simulink model "Demo_veDYNA_cs"  (Simulink 7.6)
settings: Solver=ode1  StartTime=0  StopTime=15  FixedStep=1/500  RelTol=1e-3
PreLoadFcn:
  | PreScanveDYNAPreLoadFcn(bdroot);
  | check_NUTS_defined;
  | 
  | assignin('base',['model_closed_' bdroot],false);
PostLoadFcn:
  | PreScanveDYNAPostLoadFcn(bdroot);
  | 
InitFcn:
  | vdy_SetExternalInputSource('ManLongCtrl',1,'Brake','other');
  | vdy_SetExternalInputSource('ManLongCtrl',1,'EngineTorque','other');
  | vdy_SetExternalInputSource('ManLatCtrl',1,'Steering','other');
  | 
  | PreScanveDYNAInitFcn(bdroot);
  | PreScanExperimentInitFcn(bdroot)
StopFcn:
  | PreScanExperimentStopFcn(bdroot)
undefined symbols (not defined in the file): at_period, CPT, vm_at_pulsewidth, vm_driver_dflt_gain, x_ini_VRML, y_ini_VRML, z_ini_VRML
libraries: dyna_cpt_lib x93, simulink x16, simulink_extras x14, PreScanSimulinkLibrary x6, anilib x3, dyna_lib x3, dyna_manctrl_lib x2, dyna_road_lib x2, PreScanUsefulBlocks x1, dyna_io_lib x1, dyna_demo_lib x1, dyna_usr_maneuver_states_lib x1
(part 6 of 8)

== system Demo_veDYNA_cs/Vedyna_Vehicle/CPT_MDL/MDL_SW/GearCtrl/System Instance 1 ==
  Gear [1,..,4] : Subsystem
      mask Display: disp('Input switch: value(1), table(2), io(3), other(4) [1,..,4]')
  GearMode [0,1] : Subsystem
      mask Display: disp('Input switch: internal(0), external(1) [0,1]')
  HCI [1,..,n] : Subsystem
      mask Display: disp('HCI switch [1,..,n]')
  UpShiftRequest [1,..,4] : Subsystem
      mask Display: disp('Input switch: value(1), table(2), io(3), other(4) [1,..,4]')

== system Demo_veDYNA_cs/Vedyna_Vehicle/CPT_MDL/MDL_SW/ManLatCtrl/System Instance 1 ==
  Curvature [1,..,4] : Subsystem
      mask Display: disp('Input switch: value(1), table(2), io(3), other(4) [1,..,4]')
  LatManMode [0,1,2] : Subsystem
      mask Display: disp('Input switch: internal(0), ext. steering(1), ext. curvature(2) [0,1,2]')
  Steering [1,..,4] : Subsystem
      mask Display: disp('Input switch: value(1), table(2), io(3), other(4) [1,..,4]')

== system Demo_veDYNA_cs/Vedyna_Vehicle/CPT_MDL/MDL_SW/ManLongCtrl/System Instance 1 ==
  AccelerationY [1,..,4] : Subsystem
      mask Display: disp('Input switch: value(1), table(2), io(3), other(4) [1,..,4]')
  Brake [1,..,4] : Subsystem
      mask Display: disp('Input switch: value(1), table(2), io(3), other(4) [1,..,4]')
  EngineTorque [1,..,4] : Subsystem
      mask Display: disp('Input switch: value(1), table(2), io(3), other(4) [1,..,4]')
  LongManMode [0,1,2] : Subsystem
      mask Display: disp('Input switch: internal(0), ext. throttle/brake(1), ext. speed(2) [0,1,2]')
  Speed [1,..,4] : Subsystem
      mask Display: disp('Input switch: value(1), table(2), io(3), other(4) [1,..,4]')
  Throttle [1,..,4] : Subsystem
      mask Display: disp('Input switch: value(1), table(2), io(3), other(4) [1,..,4]')

== system Demo_veDYNA_cs/Vedyna_Vehicle/CPT_MDL/MDL_SW/ManSchedule/System Instance 1 ==
  HCI [1,..,n] : Subsystem
      mask Display: disp('HCI switch [1,..,n]')

== system Demo_veDYNA_cs/Vedyna_Vehicle/CPT_MDL/MDL_SW/ManSchedule/System Instance 2 ==
  HCI [1,..,n] : Subsystem
      mask Display: disp('HCI switch [1,..,n]')

== system Demo_veDYNA_cs/Vedyna_Vehicle/CPT_MDL/MDL_SW/ManSchedule/System Instance 3 ==
  HCI [1,..,n] : Subsystem
      mask Display: disp('HCI switch [1,..,n]')

== system Demo_veDYNA_cs/Vedyna_Vehicle/CPT_MDL/MDL_SW/Road/System Instance 1 ==
  HCI [1,..,n] : Subsystem
      mask Display: disp('HCI switch [1,..,n]')

== system Demo_veDYNA_cs/Vedyna_Vehicle/CPT_MDL/MDL_SW/Simctrl/System Instance 1 ==
  Reset [0,1] : Subsystem
      mask Display: disp('Reset switch: 0/1 [0,1]')
  Suspend [0,1] : Subsystem
      mask Display: disp('Suspend switch: 0/1 [0,1]')

== system Demo_veDYNA_cs/Vedyna_Vehicle/CPT_MDL/MDL_SW/Tmeasy/System Instance 1 ==
  HCI [1,..,n] : Subsystem
      mask Display: disp('HCI switch [1,..,n]')
  RoadMueScale [1,..,4] : Subsystem
      mask Display: disp('Input switch: value(1), table(2), io(3), other(4) [1,..,4]')

== system Demo_veDYNA_cs/Vedyna_Vehicle/CPT_MDL/MDL_SW/Tmeasy/System Instance 2 ==
  HCI [1,..,n] : Subsystem
      mask Display: disp('HCI switch [1,..,n]')
  RoadMueScale [1,..,4] : Subsystem
      mask Display: disp('Input switch: value(1), table(2), io(3), other(4) [1,..,4]')

== system Demo_veDYNA_cs/Vedyna_Vehicle/CPT_MDL/MDL_SW/Tmeasy/System Instance 3 ==
  HCI [1,..,n] : Subsystem
      mask Display: disp('HCI switch [1,..,n]')
  RoadMueScale [1,..,4] : Subsystem
      mask Display: disp('Input switch: value(1), table(2), io(3), other(4) [1,..,4]')

== system Demo_veDYNA_cs/Vedyna_Vehicle/CPT_MDL/MDL_SW/Tmeasy/System Instance 4 ==
  HCI [1,..,n] : Subsystem
      mask Display: disp('HCI switch [1,..,n]')
  RoadMueScale [1,..,4] : Subsystem
      mask Display: disp('Input switch: value(1), table(2), io(3), other(4) [1,..,4]')

== system Demo_veDYNA_cs/Vedyna_Vehicle/CPT_MDL/MDL_SW/Tmeasy/System Instance 5 ==
  HCI [1,..,n] : Subsystem
      mask Display: disp('HCI switch [1,..,n]')
  RoadMueScale [1,..,4] : Subsystem
      mask Display: disp('Input switch: value(1), table(2), io(3), other(4) [1,..,4]')

== system Demo_veDYNA_cs/Vedyna_Vehicle/CPT_MDL/MDL_SW/Tmeasy/System Instance 6 ==
  HCI [1,..,n] : Subsystem
      mask Display: disp('HCI switch [1,..,n]')
  RoadMueScale [1,..,4] : Subsystem
      mask Display: disp('Input switch: value(1), table(2), io(3), other(4) [1,..,4]')

== system Demo_veDYNA_cs/Vedyna_Vehicle/CPT_MDL/MDL_SW/Tmeasy/System Instance 7 ==
  HCI [1,..,n] : Subsystem
      mask Display: disp('HCI switch [1,..,n]')
  RoadMueScale [1,..,4] : Subsystem
      mask Display: disp('Input switch: value(1), table(2), io(3), other(4) [1,..,4]')

== system Demo_veDYNA_cs/Vedyna_Vehicle/CPT_MDL/MDL_SW/Tmeasy/System Instance 8 ==
  HCI [1,..,n] : Subsystem
      mask Display: disp('HCI switch [1,..,n]')
  RoadMueScale [1,..,4] : Subsystem
      mask Display: disp('Input switch: value(1), table(2), io(3), other(4) [1,..,4]')

== system Demo_veDYNA_cs/Vedyna_Vehicle/CPT_MDL/MDL_SW/Vehicle/System Instance 1 ==
  HCI [1,..,n] : Subsystem
      mask Display: disp('HCI switch [1,..,n]')

== system Demo_veDYNA_cs/Vedyna_Vehicle/CPT_MDL/MDL_SW/Wheel/System Instance 1 ==
  HCI [1,..,n] : Subsystem
      mask Display: disp('HCI switch [1,..,n]')
  pbrm [1,..,4] : Subsystem
      mask Display: disp('Input switch: value(1), table(2), io(3), other(4) [1,..,4]')

== system Demo_veDYNA_cs/Vedyna_Vehicle/CPT_MDL/MDL_SW/Wheel/System Instance 2 ==
  HCI [1,..,n] : Subsystem
      mask Display: disp('HCI switch [1,..,n]')
  pbrm [1,..,4] : Subsystem
      mask Display: disp('Input switch: value(1), table(2), io(3), other(4) [1,..,4]')

== system Demo_veDYNA_cs/Vedyna_Vehicle/CPT_MDL/MDL_SW/Wheel/System Instance 3 ==
  HCI [1,..,n] : Subsystem
      mask Display: disp('HCI switch [1,..,n]')
  pbrm [1,..,4] : Subsystem
      mask Display: disp('Input switch: value(1), table(2), io(3), other(4) [1,..,4]')

== system Demo_veDYNA_cs/Vedyna_Vehicle/CPT_MDL/MDL_SW/Wheel/System Instance 4 ==
  HCI [1,..,n] : Subsystem
      mask Display: disp('HCI switch [1,..,n]')
  pbrm [1,..,4] : Subsystem
      mask Display: disp('Input switch: value(1), table(2), io(3), other(4) [1,..,4]')

== system Demo_veDYNA_cs/Vedyna_Vehicle/CPT_MDL/MDL_SW/Wheel/System Instance 5 ==
  HCI [1,..,n] : Subsystem
      mask Display: disp('HCI switch [1,..,n]')
  pbrm [1,..,4] : Subsystem
      mask Display: disp('Input switch: value(1), table(2), io(3), other(4) [1,..,4]')

== system Demo_veDYNA_cs/Vedyna_Vehicle/CPT_MDL/MDL_SW/Wheel/System Instance 6 ==
  HCI [1,..,n] : Subsystem
      mask Display: disp('HCI switch [1,..,n]')
  pbrm [1,..,4] : Subsystem
      mask Display: disp('Input switch: value(1), table(2), io(3), other(4) [1,..,4]')

== system Demo_veDYNA_cs/Vedyna_Vehicle/CPT_MDL/MDL_SW/Wheel/System Instance 7 ==
  HCI [1,..,n] : Subsystem
      mask Display: disp('HCI switch [1,..,n]')
  pbrm [1,..,4] : Subsystem
      mask Display: disp('Input switch: value(1), table(2), io(3), other(4) [1,..,4]')

== system Demo_veDYNA_cs/Vedyna_Vehicle/CPT_MDL/MDL_SW/Wheel/System Instance 8 ==
  HCI [1,..,n] : Subsystem
      mask Display: disp('HCI switch [1,..,n]')
  pbrm [1,..,4] : Subsystem
      mask Display: disp('Input switch: value(1), table(2), io(3), other(4) [1,..,4]')

== system Demo_veDYNA_cs/Vedyna_Vehicle/vdy_mdl/Maneuver Control/Maneuver Controller Inputs/Clutch Control Inputs ==
  Ground : Ground
  Ground1 : Ground
  Mux : Mux  Inputs=2
  PAR_ClutchCtrl_1_Clutch : dyna_cpt_lib/CPT_MDL_PAR_ACCESS  Tag=vedynaCPT_MDL_PAR_ACCESS  component=ClutchCtrl  system_inst=1  parameter=Clutch
  SW_ClutchCtrl_1_ClutchMode : dyna_cpt_lib/CPT_MDL_SW_ACCESS  Tag=vedynaCPT_MDL_HCI_ACCESS  component=ClutchCtrl  system_inst=1  parameter=ClutchMode
  Scale to [0..1] : Gain  Gain=0.01  SaturateOnIntegerOverflow=on  OutDataTypeStr=Inherit: Same as input  ParamDataTypeStr=Inherit: Same as input
  Clutch Control Inputs : Outport
  wires:
  Scale to [0..1]/1 -> Mux/2
  PAR_ClutchCtrl_1_Clutch/1 -> Scale to [0..1]/1
  Ground1/1 -> PAR_ClutchCtrl_1_Clutch/1
  Ground/1 -> PAR_ClutchCtrl_1_Clutch/2
  SW_ClutchCtrl_1_ClutchMode/1 -> Mux/1
  Mux/1 -> Clutch Control Inputs/1

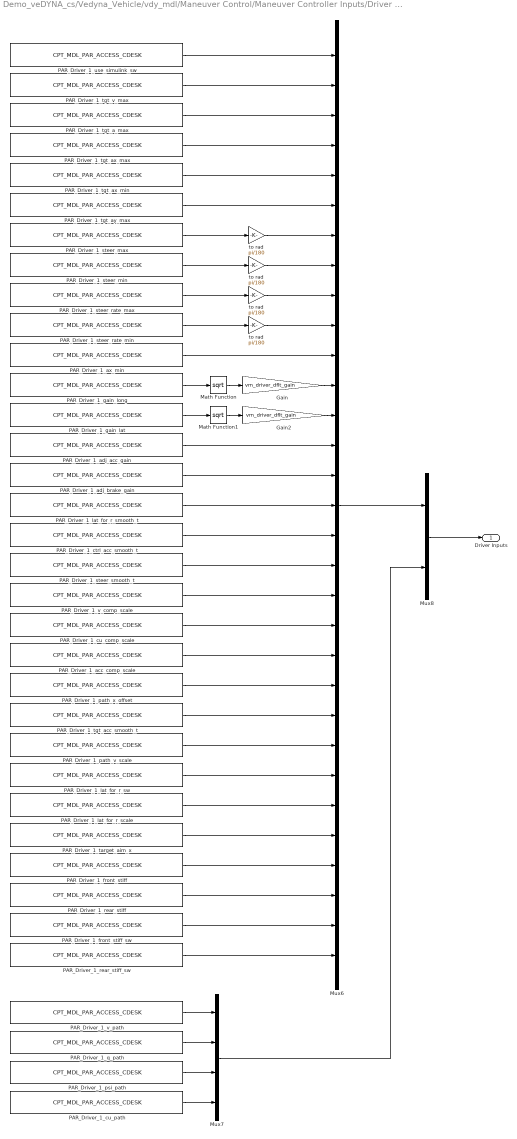
== system Demo_veDYNA_cs/Vedyna_Vehicle/vdy_mdl/Maneuver Control/Maneuver Controller Inputs/Driver Inputs ==
  Gain : Gain  Gain=vm_driver_dflt_gain  SaturateOnIntegerOverflow=on  OutDataTypeStr=Inherit: Same as input  ParamDataTypeStr=Inherit: Same as input
  Gain2 : Gain  Gain=vm_driver_dflt_gain  SaturateOnIntegerOverflow=on  OutDataTypeStr=Inherit: Same as input  ParamDataTypeStr=Inherit: Same as input
  Math Function : Math  Operator=sqrt  SaturateOnIntegerOverflow=on
  Math Function1 : Math  Operator=sqrt  SaturateOnIntegerOverflow=on
  Mux6 : Mux  Inputs=31
  Mux7 : Mux
  Mux8 : Mux  Inputs=2
  PAR_Driver_1_acc_comp_scale : dyna_cpt_lib/CPT_MDL_PAR_ACCESS_CDESK  Tag=vedynaCPT_MDL_PAR_ACCESS  component=Driver  system_inst=1  parameter=acc_comp_scale
  PAR_Driver_1_adj_acc_gain : dyna_cpt_lib/CPT_MDL_PAR_ACCESS_CDESK  Tag=vedynaCPT_MDL_PAR_ACCESS  component=Driver  system_inst=1  parameter=adj_acc_gain
  PAR_Driver_1_adj_brake_gain : dyna_cpt_lib/CPT_MDL_PAR_ACCESS_CDESK  Tag=vedynaCPT_MDL_PAR_ACCESS  component=Driver  system_inst=1  parameter=adj_brake_gain
  PAR_Driver_1_ax_min : dyna_cpt_lib/CPT_MDL_PAR_ACCESS_CDESK  Tag=vedynaCPT_MDL_PAR_ACCESS  component=Driver  system_inst=1  parameter=ax_min
  PAR_Driver_1_ctrl_acc_smooth_t : dyna_cpt_lib/CPT_MDL_PAR_ACCESS_CDESK  Tag=vedynaCPT_MDL_PAR_ACCESS  component=Driver  system_inst=1  parameter=ctrl_acc_smooth_t
  PAR_Driver_1_cu_comp_scale : dyna_cpt_lib/CPT_MDL_PAR_ACCESS_CDESK  Tag=vedynaCPT_MDL_PAR_ACCESS  component=Driver  system_inst=1  parameter=cu_comp_scale
  PAR_Driver_1_cu_path : dyna_cpt_lib/CPT_MDL_PAR_ACCESS_CDESK  Tag=vedynaCPT_MDL_PAR_ACCESS  component=Driver  system_inst=1  parameter=cu_path
  PAR_Driver_1_front_stiff : dyna_cpt_lib/CPT_MDL_PAR_ACCESS_CDESK  Tag=vedynaCPT_MDL_PAR_ACCESS  component=Driver  system_inst=1  parameter=front_stiff
  PAR_Driver_1_front_stiff_sw : dyna_cpt_lib/CPT_MDL_PAR_ACCESS_CDESK  Tag=vedynaCPT_MDL_PAR_ACCESS  component=Driver  system_inst=1  parameter=front_stiff_sw
  PAR_Driver_1_gain_lat : dyna_cpt_lib/CPT_MDL_PAR_ACCESS_CDESK  Tag=vedynaCPT_MDL_PAR_ACCESS  component=Driver  system_inst=1  parameter=gain_lat
  PAR_Driver_1_gain_long : dyna_cpt_lib/CPT_MDL_PAR_ACCESS_CDESK  Tag=vedynaCPT_MDL_PAR_ACCESS  component=Driver  system_inst=1  parameter=gain_long
  PAR_Driver_1_lat_for_r_scale : dyna_cpt_lib/CPT_MDL_PAR_ACCESS_CDESK  Tag=vedynaCPT_MDL_PAR_ACCESS  component=Driver  system_inst=1  parameter=lat_for_r_scale
  PAR_Driver_1_lat_for_r_smooth_t : dyna_cpt_lib/CPT_MDL_PAR_ACCESS_CDESK  Tag=vedynaCPT_MDL_PAR_ACCESS  component=Driver  system_inst=1  parameter=lat_for_r_smooth_t
  PAR_Driver_1_lat_for_r_sw : dyna_cpt_lib/CPT_MDL_PAR_ACCESS_CDESK  Tag=vedynaCPT_MDL_PAR_ACCESS  component=Driver  system_inst=1  parameter=lat_for_r_sw
  PAR_Driver_1_path_v_scale : dyna_cpt_lib/CPT_MDL_PAR_ACCESS_CDESK  Tag=vedynaCPT_MDL_PAR_ACCESS  component=Driver  system_inst=1  parameter=path_v_scale
  PAR_Driver_1_path_x_offset : dyna_cpt_lib/CPT_MDL_PAR_ACCESS_CDESK  Tag=vedynaCPT_MDL_PAR_ACCESS  component=Driver  system_inst=1  parameter=path_x_offset
  PAR_Driver_1_psi_path : dyna_cpt_lib/CPT_MDL_PAR_ACCESS_CDESK  Tag=vedynaCPT_MDL_PAR_ACCESS  component=Driver  system_inst=1  parameter=psi_path
  PAR_Driver_1_q_path : dyna_cpt_lib/CPT_MDL_PAR_ACCESS_CDESK  Tag=vedynaCPT_MDL_PAR_ACCESS  component=Driver  system_inst=1  parameter=q_path
  PAR_Driver_1_rear_stiff : dyna_cpt_lib/CPT_MDL_PAR_ACCESS_CDESK  Tag=vedynaCPT_MDL_PAR_ACCESS  component=Driver  system_inst=1  parameter=rear_stiff
  PAR_Driver_1_rear_stiff_sw : dyna_cpt_lib/CPT_MDL_PAR_ACCESS_CDESK  Tag=vedynaCPT_MDL_PAR_ACCESS  component=Driver  system_inst=1  parameter=rear_stiff_sw
  PAR_Driver_1_steer_max : dyna_cpt_lib/CPT_MDL_PAR_ACCESS_CDESK  Tag=vedynaCPT_MDL_PAR_ACCESS  component=Driver  system_inst=1  parameter=steer_max
  PAR_Driver_1_steer_min : dyna_cpt_lib/CPT_MDL_PAR_ACCESS_CDESK  Tag=vedynaCPT_MDL_PAR_ACCESS  component=Driver  system_inst=1  parameter=steer_min
  PAR_Driver_1_steer_rate_max : dyna_cpt_lib/CPT_MDL_PAR_ACCESS_CDESK  Tag=vedynaCPT_MDL_PAR_ACCESS  component=Driver  system_inst=1  parameter=steer_rate_max
  PAR_Driver_1_steer_rate_min : dyna_cpt_lib/CPT_MDL_PAR_ACCESS_CDESK  Tag=vedynaCPT_MDL_PAR_ACCESS  component=Driver  system_inst=1  parameter=steer_rate_min
  PAR_Driver_1_steer_smooth_t : dyna_cpt_lib/CPT_MDL_PAR_ACCESS_CDESK  Tag=vedynaCPT_MDL_PAR_ACCESS  component=Driver  system_inst=1  parameter=steer_smooth_t
  PAR_Driver_1_target_aim_x : dyna_cpt_lib/CPT_MDL_PAR_ACCESS_CDESK  Tag=vedynaCPT_MDL_PAR_ACCESS  component=Driver  system_inst=1  parameter=target_aim_x
  PAR_Driver_1_tgt_a_max : dyna_cpt_lib/CPT_MDL_PAR_ACCESS_CDESK  Tag=vedynaCPT_MDL_PAR_ACCESS  component=Driver  system_inst=1  parameter=tgt_a_max
  PAR_Driver_1_tgt_acc_smooth_t : dyna_cpt_lib/CPT_MDL_PAR_ACCESS_CDESK  Tag=vedynaCPT_MDL_PAR_ACCESS  component=Driver  system_inst=1  parameter=tgt_acc_smooth_t
  PAR_Driver_1_tgt_ax_max : dyna_cpt_lib/CPT_MDL_PAR_ACCESS_CDESK  Tag=vedynaCPT_MDL_PAR_ACCESS  component=Driver  system_inst=1  parameter=tgt_ax_max
  PAR_Driver_1_tgt_ax_min : dyna_cpt_lib/CPT_MDL_PAR_ACCESS_CDESK  Tag=vedynaCPT_MDL_PAR_ACCESS  component=Driver  system_inst=1  parameter=tgt_ax_min
  PAR_Driver_1_tgt_ay_max : dyna_cpt_lib/CPT_MDL_PAR_ACCESS_CDESK  Tag=vedynaCPT_MDL_PAR_ACCESS  component=Driver  system_inst=1  parameter=tgt_ay_max
  PAR_Driver_1_tgt_v_max : dyna_cpt_lib/CPT_MDL_PAR_ACCESS_CDESK  Tag=vedynaCPT_MDL_PAR_ACCESS  component=Driver  system_inst=1  parameter=tgt_v_max
  PAR_Driver_1_use_simulink_sw : dyna_cpt_lib/CPT_MDL_PAR_ACCESS_CDESK  Tag=vedynaCPT_MDL_PAR_ACCESS  component=Driver  system_inst=1  parameter=use_simulink_sw
  PAR_Driver_1_v_comp_scale : dyna_cpt_lib/CPT_MDL_PAR_ACCESS_CDESK  Tag=vedynaCPT_MDL_PAR_ACCESS  component=Driver  system_inst=1  parameter=v_comp_scale
  PAR_Driver_1_v_path : dyna_cpt_lib/CPT_MDL_PAR_ACCESS_CDESK  Tag=vedynaCPT_MDL_PAR_ACCESS  component=Driver  system_inst=1  parameter=v_path
  to rad : Gain  Gain=pi/180  SaturateOnIntegerOverflow=on  OutDataTypeStr=Inherit: Same as input  ParamDataTypeStr=Inherit: Same as input
  "to rad " : Gain  Gain=pi/180  SaturateOnIntegerOverflow=on  OutDataTypeStr=Inherit: Same as input  ParamDataTypeStr=Inherit: Same as input
  "to rad  " : Gain  Gain=pi/180  SaturateOnIntegerOverflow=on  OutDataTypeStr=Inherit: Same as input  ParamDataTypeStr=Inherit: Same as input
  "to rad   " : Gain  Gain=pi/180  SaturateOnIntegerOverflow=on  OutDataTypeStr=Inherit: Same as input  ParamDataTypeStr=Inherit: Same as input
  Driver Inputs : Outport
  wires:
  to rad/1 -> Mux6/7
  PAR_Driver_1_steer_max/1 -> to rad/1
  "to rad "/1 -> Mux6/8
  PAR_Driver_1_steer_min/1 -> "to rad "/1
  "to rad  "/1 -> Mux6/9
  PAR_Driver_1_steer_rate_max/1 -> "to rad  "/1
  "to rad   "/1 -> Mux6/10
  PAR_Driver_1_steer_rate_min/1 -> "to rad   "/1
  Math Function1/1 -> Gain2/1
  PAR_Driver_1_gain_lat/1 -> Math Function1/1
  Math Function/1 -> Gain/1
  PAR_Driver_1_gain_long/1 -> Math Function/1
  Gain2/1 -> Mux6/13
  Gain/1 -> Mux6/12
  Mux7/1 -> Mux8/2
  Mux8/1 -> Driver Inputs/1
  Mux6/1 -> Mux8/1
  PAR_Driver_1_cu_path/1 -> Mux7/4
  PAR_Driver_1_psi_path/1 -> Mux7/3
  PAR_Driver_1_q_path/1 -> Mux7/2
  PAR_Driver_1_v_path/1 -> Mux7/1
  PAR_Driver_1_rear_stiff_sw/1 -> Mux6/31
  PAR_Driver_1_front_stiff_sw/1 -> Mux6/30
  PAR_Driver_1_rear_stiff/1 -> Mux6/29
  PAR_Driver_1_front_stiff/1 -> Mux6/28
  PAR_Driver_1_target_aim_x/1 -> Mux6/27
  PAR_Driver_1_lat_for_r_scale/1 -> Mux6/26
  PAR_Driver_1_lat_for_r_sw/1 -> Mux6/25
  PAR_Driver_1_path_v_scale/1 -> Mux6/24
  PAR_Driver_1_tgt_acc_smooth_t/1 -> Mux6/23
  PAR_Driver_1_path_x_offset/1 -> Mux6/22
  PAR_Driver_1_acc_comp_scale/1 -> Mux6/21
  PAR_Driver_1_cu_comp_scale/1 -> Mux6/20
  PAR_Driver_1_v_comp_scale/1 -> Mux6/19
  PAR_Driver_1_steer_smooth_t/1 -> Mux6/18
  PAR_Driver_1_ctrl_acc_smooth_t/1 -> Mux6/17
  PAR_Driver_1_lat_for_r_smooth_t/1 -> Mux6/16
  PAR_Driver_1_adj_brake_gain/1 -> Mux6/15
  PAR_Driver_1_adj_acc_gain/1 -> Mux6/14
  PAR_Driver_1_ax_min/1 -> Mux6/11
  PAR_Driver_1_tgt_ay_max/1 -> Mux6/6
  PAR_Driver_1_tgt_ax_min/1 -> Mux6/5
  PAR_Driver_1_tgt_ax_max/1 -> Mux6/4
  PAR_Driver_1_tgt_a_max/1 -> Mux6/3
  PAR_Driver_1_tgt_v_max/1 -> Mux6/2
  PAR_Driver_1_use_simulink_sw/1 -> Mux6/1

== system Demo_veDYNA_cs/Vedyna_Vehicle/vdy_mdl/Maneuver Control/Maneuver Controller Inputs/Gear Control Inputs ==
  Ground{,1..3} (4 alike) : Ground
  Mux : Mux  Inputs=3
  PAR_GearCtrl_1_Gear : dyna_cpt_lib/CPT_MDL_PAR_ACCESS  Tag=vedynaCPT_MDL_PAR_ACCESS  component=GearCtrl  system_inst=1  parameter=Gear
  PAR_GearCtrl_1_UpShiftRequest : dyna_cpt_lib/CPT_MDL_PAR_ACCESS  Tag=vedynaCPT_MDL_PAR_ACCESS  component=GearCtrl  system_inst=1  parameter=UpShiftRequest
  SW_GearCtrl_1_GearMode : dyna_cpt_lib/CPT_MDL_SW_ACCESS  Tag=vedynaCPT_MDL_HCI_ACCESS  component=GearCtrl  system_inst=1  parameter=GearMode
  Gear Control Inputs : Outport
  wires:
  Ground1/1 -> PAR_GearCtrl_1_Gear/1
  Ground/1 -> PAR_GearCtrl_1_Gear/2
  SW_GearCtrl_1_GearMode/1 -> Mux/1
  PAR_GearCtrl_1_Gear/1 -> Mux/2
  PAR_GearCtrl_1_UpShiftRequest/1 -> Mux/3
  Ground3/1 -> PAR_GearCtrl_1_UpShiftRequest/1
  Ground2/1 -> PAR_GearCtrl_1_UpShiftRequest/2
  Mux/1 -> Gear Control Inputs/1

== system Demo_veDYNA_cs/Vedyna_Vehicle/vdy_mdl/Maneuver Control/Maneuver Controller Inputs/Lateral Control Inputs ==
  Ground{,1..3} (4 alike) : Ground
  Mux : Mux  Inputs=3
  PAR_ManLatCtrl_1_Curvature : dyna_cpt_lib/CPT_MDL_PAR_ACCESS  Tag=vedynaCPT_MDL_PAR_ACCESS  component=ManLatCtrl  system_inst=1  parameter=Curvature
  PAR_ManLatCtrl_1_Steering : dyna_cpt_lib/CPT_MDL_PAR_ACCESS  Tag=vedynaCPT_MDL_PAR_ACCESS  component=ManLatCtrl  system_inst=1  parameter=Steering
  SW_ManLatCtrl_1_LatManMode : dyna_cpt_lib/CPT_MDL_SW_ACCESS  Tag=vedynaCPT_MDL_HCI_ACCESS  component=ManLatCtrl  system_inst=1  parameter=LatManMode
  Scale to [rad] : Gain  Gain=pi/180  SaturateOnIntegerOverflow=on  OutDataTypeStr=Inherit: Same as input  ParamDataTypeStr=Inherit: Same as input
  Lateral Control Inputs : Outport
  wires:
  Scale to [rad]/1 -> Mux/2
  PAR_ManLatCtrl_1_Steering/1 -> Scale to [rad]/1
  SW_ManLatCtrl_1_LatManMode/1 -> Mux/1
  PAR_ManLatCtrl_1_Curvature/1 -> Mux/3
  Ground1/1 -> PAR_ManLatCtrl_1_Steering/1
  Ground/1 -> PAR_ManLatCtrl_1_Steering/2
  Ground3/1 -> PAR_ManLatCtrl_1_Curvature/1
  Ground2/1 -> PAR_ManLatCtrl_1_Curvature/2
  Mux/1 -> Lateral Control Inputs/1

== system Demo_veDYNA_cs/Vedyna_Vehicle/vdy_mdl/Maneuver Control/Maneuver Controller Inputs/Longitudinal Control Inputs ==
  Ground{,1..9} (10 alike) : Ground
  Mux : Mux  Inputs=6
  PAR_ManLongCtrl_1_AccelerationY : dyna_cpt_lib/CPT_MDL_PAR_ACCESS  Tag=vedynaCPT_MDL_PAR_ACCESS  component=ManLongCtrl  system_inst=1  parameter=AccelerationY
  PAR_ManLongCtrl_1_Brake : dyna_cpt_lib/CPT_MDL_PAR_ACCESS  Tag=vedynaCPT_MDL_PAR_ACCESS  component=ManLongCtrl  system_inst=1  parameter=Brake
  PAR_ManLongCtrl_1_EngineTorque : dyna_cpt_lib/CPT_MDL_PAR_ACCESS  Tag=vedynaCPT_MDL_PAR_ACCESS  component=ManLongCtrl  system_inst=1  parameter=EngineTorque
  PAR_ManLongCtrl_1_Speed : dyna_cpt_lib/CPT_MDL_PAR_ACCESS  Tag=vedynaCPT_MDL_PAR_ACCESS  component=ManLongCtrl  system_inst=1  parameter=Speed
  PAR_ManLongCtrl_1_Throttle : dyna_cpt_lib/CPT_MDL_PAR_ACCESS  Tag=vedynaCPT_MDL_PAR_ACCESS  component=ManLongCtrl  system_inst=1  parameter=Throttle
  SW_ManLongCtrl_1_LongManMode : dyna_cpt_lib/CPT_MDL_SW_ACCESS  Tag=vedynaCPT_MDL_HCI_ACCESS  component=ManLongCtrl  system_inst=1  parameter=LongManMode
  Scale to [0..1] : Gain  Gain=0.01  SaturateOnIntegerOverflow=on  OutDataTypeStr=Inherit: Same as input  ParamDataTypeStr=Inherit: Same as input
  Scale to [0..1]1 : Gain  Gain=0.01  SaturateOnIntegerOverflow=on  OutDataTypeStr=Inherit: Same as input  ParamDataTypeStr=Inherit: Same as input
  Scale to [m/s] : Gain  Gain=1/3.6  SaturateOnIntegerOverflow=on  OutDataTypeStr=Inherit: Same as input  ParamDataTypeStr=Inherit: Same as input
  Longitudinal Control Inputs : Outport
  wires:
  Scale to [m/s]/1 -> Mux/5
  PAR_ManLongCtrl_1_Speed/1 -> Scale to [m/s]/1
  Scale to [0..1]1/1 -> Mux/3
  PAR_ManLongCtrl_1_Brake/1 -> Scale to [0..1]1/1
  Scale to [0..1]/1 -> Mux/2
  PAR_ManLongCtrl_1_Throttle/1 -> Scale to [0..1]/1
  Ground1/1 -> PAR_ManLongCtrl_1_Throttle/1
  Ground/1 -> PAR_ManLongCtrl_1_Throttle/2
  SW_ManLongCtrl_1_LongManMode/1 -> Mux/1
  PAR_ManLongCtrl_1_AccelerationY/1 -> Mux/4
  PAR_ManLongCtrl_1_EngineTorque/1 -> Mux/6
  Ground9/1 -> PAR_ManLongCtrl_1_EngineTorque/1
  Ground8/1 -> PAR_ManLongCtrl_1_EngineTorque/2
  Ground7/1 -> PAR_ManLongCtrl_1_Speed/1
  Ground6/1 -> PAR_ManLongCtrl_1_Speed/2
  Ground5/1 -> PAR_ManLongCtrl_1_AccelerationY/1
  Ground4/1 -> PAR_ManLongCtrl_1_AccelerationY/2
  Ground3/1 -> PAR_ManLongCtrl_1_Brake/1
  Ground2/1 -> PAR_ManLongCtrl_1_Brake/2
  Mux/1 -> Longitudinal Control Inputs/1

== system Demo_veDYNA_cs/Vedyna_Vehicle/vdy_mdl/Road/veDYNA Road Subsystem/HCI Switch ==
  SW_Road_1_HCI : dyna_cpt_lib/CPT_MDL_HCI_SW_ACCESS  Tag=vedynaCPT_MDL_HCI_SW_ACCESS  component=Road  system_inst=1  parameter=HCI
  HCI Switch : Outport
  wires:
  SW_Road_1_HCI/1 -> HCI Switch/1

== system Demo_veDYNA_cs/Vedyna_Vehicle/vdy_mdl/Vehicle System/veDYNA Vehicle Subsystem/Brake System ==
  note: COPYRIGHT 2004 by TESIS DYNAware GmbH
  note: veDYNA Vehicle Brake System
  SyncIn : Inport
  I/O Vector : Inport  Port=2
  Brake Pedal Position : Inport  Port=3
  Configurable Subsystem : Subsystem  BlockChoice=veDYNA Brake Hydraulics
      settings: AttributesFormatString=%<BlockChoice>  MemberBlocks=User Defined Brake Hydraulics,veDYNA Brake Hydraulics,veDYNA Brake Hydraulics Trailer
      settings: TemplateBlock=|
      | dyna_brakehydraulics_lib/Configurable
      | Subsystem
  Constant{,1..5} (6 alike) : Constant  Value=0
  HCI Switch : Subsystem
  Mux1 : Mux  Inputs=6
  PAR_Wheel_1_pbrm : dyna_cpt_lib/CPT_MDL_PAR_ACCESS  Tag=vedynaCPT_MDL_PAR_ACCESS  component=Wheel  system_inst=1  parameter=pbrm
  PAR_Wheel_2_pbrm : dyna_cpt_lib/CPT_MDL_PAR_ACCESS  Tag=vedynaCPT_MDL_PAR_ACCESS  component=Wheel  system_inst=2  parameter=pbrm
  PAR_Wheel_3_pbrm : dyna_cpt_lib/CPT_MDL_PAR_ACCESS  Tag=vedynaCPT_MDL_PAR_ACCESS  component=Wheel  system_inst=3  parameter=pbrm
  PAR_Wheel_4_pbrm : dyna_cpt_lib/CPT_MDL_PAR_ACCESS  Tag=vedynaCPT_MDL_PAR_ACCESS  component=Wheel  system_inst=4  parameter=pbrm
  PAR_Wheel_5_pbrm : dyna_cpt_lib/CPT_MDL_PAR_ACCESS  Tag=vedynaCPT_MDL_PAR_ACCESS  component=Wheel  system_inst=5  parameter=pbrm
  PAR_Wheel_6_pbrm : dyna_cpt_lib/CPT_MDL_PAR_ACCESS  Tag=vedynaCPT_MDL_PAR_ACCESS  component=Wheel  system_inst=6  parameter=pbrm
  Terminator10 : Terminator
  Terminator4 : Terminator
  Brake Hydraulics Info : Outport
  SyncOut : Outport  Port=2
  Master Cylinder Pressure : Outport  Port=3
  Wheel Cylinder Pressures : Outport  Port=4
  tag scope: pb=global, pbmax=global
  wires:
  Configurable Subsystem/11(Wheel 8 Cylinder Pressure) -> Terminator10/1
  Configurable Subsystem/10(Wheel 7 Cylinder Pressure) -> Terminator4/1
  I/O Vector/1 -> Configurable Subsystem/2(I/O Vector)
  PAR_Wheel_2_pbrm/1 -> Mux1/2
  PAR_Wheel_3_pbrm/1 -> Mux1/3
  PAR_Wheel_4_pbrm/1 -> Mux1/4
  Mux1/1 -> Wheel Cylinder Pressures/1
  SyncIn/1 -> Configurable Subsystem/3(SyncIn)
  Brake Pedal Position/1 -> Configurable Subsystem/1(Brake Pedal Position)
  PAR_Wheel_1_pbrm/1 -> Mux1/1
  Configurable Subsystem/1(SyncOut) -> SyncOut/1
  Configurable Subsystem/2(BrkHyd Info) -> Brake Hydraulics Info/1, [pbmax]
  Configurable Subsystem/3(Master Cylinder Pressure) -> Master Cylinder Pressure/1, [pb]
  PAR_Wheel_5_pbrm/1 -> Mux1/5
  PAR_Wheel_6_pbrm/1 -> Mux1/6
  HCI Switch/1(HCI Switch) -> Configurable Subsystem/4(HCI Switch)
  Constant/1 -> PAR_Wheel_1_pbrm/1
  Configurable Subsystem/4(Wheel 1 Cylinder Pressure) -> PAR_Wheel_1_pbrm/2
  Configurable Subsystem/5(Wheel 2 Cylinder Pressure) -> PAR_Wheel_2_pbrm/2
  Configurable Subsystem/6(Wheel 3 Cylinder Pressure) -> PAR_Wheel_3_pbrm/2
  Configurable Subsystem/7(Wheel 4 Cylinder Pressure) -> PAR_Wheel_4_pbrm/2
  Configurable Subsystem/8(Wheel 5 Cylinder Pressure) -> PAR_Wheel_5_pbrm/2
  Configurable Subsystem/9(Wheel 6 Cylinder Pressure) -> PAR_Wheel_6_pbrm/2
  Constant1/1 -> PAR_Wheel_2_pbrm/1
  Constant2/1 -> PAR_Wheel_3_pbrm/1
  Constant3/1 -> PAR_Wheel_4_pbrm/1
  Constant4/1 -> PAR_Wheel_5_pbrm/1
  Constant5/1 -> PAR_Wheel_6_pbrm/1

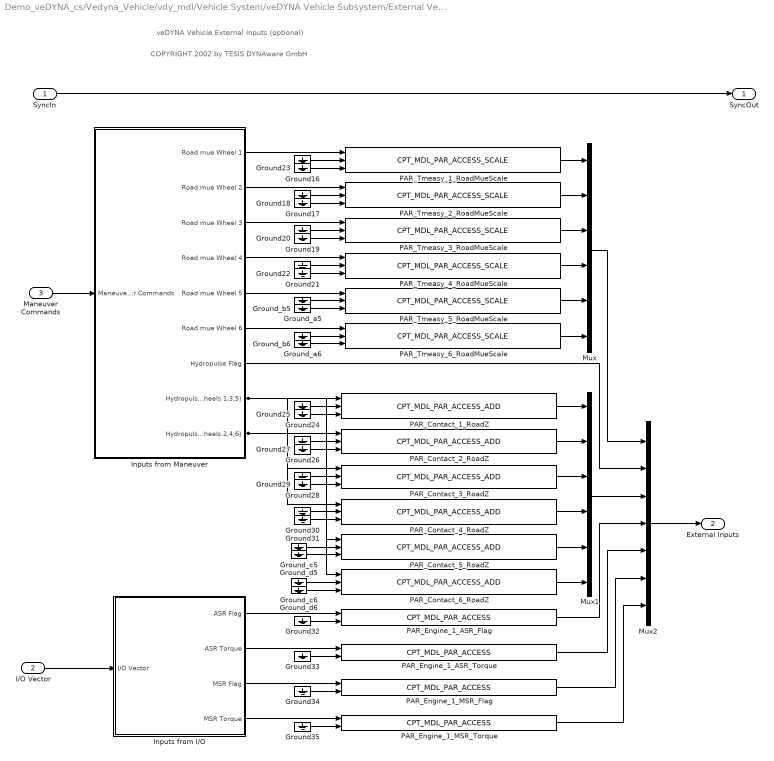
== system Demo_veDYNA_cs/Vedyna_Vehicle/vdy_mdl/Vehicle System/veDYNA Vehicle Subsystem/External Vehicle Inputs (from I/O) ==
  note: COPYRIGHT 2002 by TESIS DYNAware GmbH
  note: veDYNA Vehicle External Inputs (optional)
  SyncIn : Inport
  I/O Vector : Inport  Port=2
  Maneuver Commands : Inport  Port=3
  Ground{16..35} (20 alike) : Ground
  Ground_a5 : Ground
  Ground_a6 : Ground
  Ground_b5 : Ground
  Ground_b6 : Ground
  Ground_c5 : Ground
  Ground_c6 : Ground
  Ground_d5 : Ground
  Ground_d6 : Ground
  Inputs from I/O : Subsystem
  Inputs from Maneuver : Subsystem
  Mux : Mux  Inputs=6
  Mux1 : Mux  Inputs=6
  Mux2 : Mux  Inputs=7
  PAR_Contact_1_RoadZ : dyna_cpt_lib/CPT_MDL_PAR_ACCESS_ADD  Tag=vedynaCPT_MDL_PAR_ACCESS  component=Contact  system_inst=1  parameter=RoadZ
  PAR_Contact_2_RoadZ : dyna_cpt_lib/CPT_MDL_PAR_ACCESS_ADD  Tag=vedynaCPT_MDL_PAR_ACCESS  component=Contact  system_inst=2  parameter=RoadZ
  PAR_Contact_3_RoadZ : dyna_cpt_lib/CPT_MDL_PAR_ACCESS_ADD  Tag=vedynaCPT_MDL_PAR_ACCESS  component=Contact  system_inst=3  parameter=RoadZ
  PAR_Contact_4_RoadZ : dyna_cpt_lib/CPT_MDL_PAR_ACCESS_ADD  Tag=vedynaCPT_MDL_PAR_ACCESS  component=Contact  system_inst=4  parameter=RoadZ
  PAR_Contact_5_RoadZ : dyna_cpt_lib/CPT_MDL_PAR_ACCESS_ADD  Tag=vedynaCPT_MDL_PAR_ACCESS  component=Contact  system_inst=5  parameter=RoadZ
  PAR_Contact_6_RoadZ : dyna_cpt_lib/CPT_MDL_PAR_ACCESS_ADD  Tag=vedynaCPT_MDL_PAR_ACCESS  component=Contact  system_inst=6  parameter=RoadZ
  PAR_Engine_1_ASR_Flag : dyna_cpt_lib/CPT_MDL_PAR_ACCESS  Tag=vedynaCPT_MDL_PAR_ACCESS  component=Engine  system_inst=1  parameter=ASR_Flag
  PAR_Engine_1_ASR_Torque : dyna_cpt_lib/CPT_MDL_PAR_ACCESS  Tag=vedynaCPT_MDL_PAR_ACCESS  component=Engine  system_inst=1  parameter=ASR_Torque
  PAR_Engine_1_MSR_Flag : dyna_cpt_lib/CPT_MDL_PAR_ACCESS  Tag=vedynaCPT_MDL_PAR_ACCESS  component=Engine  system_inst=1  parameter=MSR_Flag
  PAR_Engine_1_MSR_Torque : dyna_cpt_lib/CPT_MDL_PAR_ACCESS  Tag=vedynaCPT_MDL_PAR_ACCESS  component=Engine  system_inst=1  parameter=MSR_Torque
  PAR_Tmeasy_1_RoadMueScale : dyna_cpt_lib/CPT_MDL_PAR_ACCESS_SCALE  Tag=vedynaCPT_MDL_PAR_ACCESS  component=Tmeasy  system_inst=1  parameter=RoadMueScale
  PAR_Tmeasy_2_RoadMueScale : dyna_cpt_lib/CPT_MDL_PAR_ACCESS_SCALE  Tag=vedynaCPT_MDL_PAR_ACCESS  component=Tmeasy  system_inst=2  parameter=RoadMueScale
  PAR_Tmeasy_3_RoadMueScale : dyna_cpt_lib/CPT_MDL_PAR_ACCESS_SCALE  Tag=vedynaCPT_MDL_PAR_ACCESS  component=Tmeasy  system_inst=3  parameter=RoadMueScale
  PAR_Tmeasy_4_RoadMueScale : dyna_cpt_lib/CPT_MDL_PAR_ACCESS_SCALE  Tag=vedynaCPT_MDL_PAR_ACCESS  component=Tmeasy  system_inst=4  parameter=RoadMueScale
  PAR_Tmeasy_5_RoadMueScale : dyna_cpt_lib/CPT_MDL_PAR_ACCESS_SCALE  Tag=vedynaCPT_MDL_PAR_ACCESS  component=Tmeasy  system_inst=5  parameter=RoadMueScale
  PAR_Tmeasy_6_RoadMueScale : dyna_cpt_lib/CPT_MDL_PAR_ACCESS_SCALE  Tag=vedynaCPT_MDL_PAR_ACCESS  component=Tmeasy  system_inst=6  parameter=RoadMueScale
  SyncOut : Outport
  External Inputs : Outport  Port=2
  wires:
  PAR_Contact_6_RoadZ/1 -> Mux1/6
  Ground_d6/1 -> PAR_Contact_6_RoadZ/3
  Ground_c6/1 -> PAR_Contact_6_RoadZ/2
  PAR_Contact_5_RoadZ/1 -> Mux1/5
  Ground_d5/1 -> PAR_Contact_5_RoadZ/3
  Ground_c5/1 -> PAR_Contact_5_RoadZ/2
  Inputs from Maneuver/9(Hydropulse Right (Wheels 2,4,6)) -> PAR_Contact_6_RoadZ/1, PAR_Contact_4_RoadZ/1, PAR_Contact_2_RoadZ/1
  Inputs from Maneuver/8(Hydropulse Left (Wheels 1,3,5)) -> PAR_Contact_5_RoadZ/1, PAR_Contact_3_RoadZ/1, PAR_Contact_1_RoadZ/1
  PAR_Tmeasy_6_RoadMueScale/1 -> Mux/6
  Inputs from Maneuver/6(Road mue Wheel 6) -> PAR_Tmeasy_6_RoadMueScale/1
  Ground_b6/1 -> PAR_Tmeasy_6_RoadMueScale/3
  Ground_a6/1 -> PAR_Tmeasy_6_RoadMueScale/2
  PAR_Tmeasy_5_RoadMueScale/1 -> Mux/5
  Inputs from Maneuver/5(Road mue Wheel 5) -> PAR_Tmeasy_5_RoadMueScale/1
  Ground_b5/1 -> PAR_Tmeasy_5_RoadMueScale/3
  Ground_a5/1 -> PAR_Tmeasy_5_RoadMueScale/2
  Ground16/1 -> PAR_Tmeasy_1_RoadMueScale/2
  Ground17/1 -> PAR_Tmeasy_2_RoadMueScale/2
  Ground18/1 -> PAR_Tmeasy_2_RoadMueScale/3
  Ground19/1 -> PAR_Tmeasy_3_RoadMueScale/2
  Ground20/1 -> PAR_Tmeasy_3_RoadMueScale/3
  Ground21/1 -> PAR_Tmeasy_4_RoadMueScale/2
  Ground22/1 -> PAR_Tmeasy_4_RoadMueScale/3
  Ground23/1 -> PAR_Tmeasy_1_RoadMueScale/3
  Ground24/1 -> PAR_Contact_1_RoadZ/2
  Ground25/1 -> PAR_Contact_1_RoadZ/3
  Ground26/1 -> PAR_Contact_2_RoadZ/2
  Ground27/1 -> PAR_Contact_2_RoadZ/3
  Ground28/1 -> PAR_Contact_3_RoadZ/2
  Ground29/1 -> PAR_Contact_3_RoadZ/3
  Ground30/1 -> PAR_Contact_4_RoadZ/2
  Ground31/1 -> PAR_Contact_4_RoadZ/3
  PAR_Tmeasy_1_RoadMueScale/1 -> Mux/1
  PAR_Tmeasy_2_RoadMueScale/1 -> Mux/2
  PAR_Contact_1_RoadZ/1 -> Mux1/1
  PAR_Contact_2_RoadZ/1 -> Mux1/2
  Inputs from Maneuver/1(Road mue Wheel 1) -> PAR_Tmeasy_1_RoadMueScale/1
  Inputs from Maneuver/2(Road mue Wheel 2) -> PAR_Tmeasy_2_RoadMueScale/1
  Inputs from Maneuver/3(Road mue Wheel 3) -> PAR_Tmeasy_3_RoadMueScale/1
  Inputs from Maneuver/4(Road mue Wheel 4) -> PAR_Tmeasy_4_RoadMueScale/1
  Maneuver Commands/1 -> Inputs from Maneuver/1(Maneuver Commands)
  SyncIn/1 -> SyncOut/1
  Ground32/1 -> PAR_Engine_1_ASR_Flag/2
  Ground33/1 -> PAR_Engine_1_ASR_Torque/2
  Ground34/1 -> PAR_Engine_1_MSR_Flag/2
  Ground35/1 -> PAR_Engine_1_MSR_Torque/2
  I/O Vector/1 -> Inputs from I/O/1(I/O Vector)
  Inputs from I/O/1(ASR Flag) -> PAR_Engine_1_ASR_Flag/1
  Inputs from I/O/2(ASR Torque) -> PAR_Engine_1_ASR_Torque/1
  Inputs from I/O/3(MSR Flag) -> PAR_Engine_1_MSR_Flag/1
  Inputs from I/O/4(MSR Torque) -> PAR_Engine_1_MSR_Torque/1
  PAR_Tmeasy_3_RoadMueScale/1 -> Mux/3
  PAR_Tmeasy_4_RoadMueScale/1 -> Mux/4
  PAR_Contact_3_RoadZ/1 -> Mux1/3
  PAR_Contact_4_RoadZ/1 -> Mux1/4
  Mux/1 -> Mux2/1
  Mux2/1 -> External Inputs/1
  Inputs from Maneuver/7(Hydropulse Flag) -> Mux2/2
  Mux1/1 -> Mux2/3
  PAR_Engine_1_ASR_Flag/1 -> Mux2/4
  PAR_Engine_1_ASR_Torque/1 -> Mux2/5
  PAR_Engine_1_MSR_Flag/1 -> Mux2/6
  PAR_Engine_1_MSR_Torque/1 -> Mux2/7

== system Demo_veDYNA_cs/Vedyna_Vehicle/vdy_mdl/Vehicle System/veDYNA Vehicle Subsystem/HCI Switches ==
  Mux : Mux  Inputs=28
  SW_Chassis_1_HCI : dyna_cpt_lib/CPT_MDL_HCI_SW_ACCESS  Tag=vedynaCPT_MDL_HCI_SW_ACCESS  component=Chassis  system_inst=1  parameter=HCI
  SW_Driveline_1_HCI : dyna_cpt_lib/CPT_MDL_HCI_SW_ACCESS  Tag=vedynaCPT_MDL_HCI_SW_ACCESS  component=Driveline  system_inst=1  parameter=HCI
  SW_Engine_1_HCI : dyna_cpt_lib/CPT_MDL_HCI_SW_ACCESS  Tag=vedynaCPT_MDL_HCI_SW_ACCESS  component=Engine  system_inst=1  parameter=HCI
  SW_Tmeasy_1_HCI : dyna_cpt_lib/CPT_MDL_HCI_SW_ACCESS  Tag=vedynaCPT_MDL_HCI_SW_ACCESS  component=Tmeasy  system_inst=1  parameter=HCI
  SW_Tmeasy_2_HCI : dyna_cpt_lib/CPT_MDL_HCI_SW_ACCESS  Tag=vedynaCPT_MDL_HCI_SW_ACCESS  component=Tmeasy  system_inst=2  parameter=HCI
  SW_Tmeasy_3_HCI : dyna_cpt_lib/CPT_MDL_HCI_SW_ACCESS  Tag=vedynaCPT_MDL_HCI_SW_ACCESS  component=Tmeasy  system_inst=3  parameter=HCI
  SW_Tmeasy_4_HCI : dyna_cpt_lib/CPT_MDL_HCI_SW_ACCESS  Tag=vedynaCPT_MDL_HCI_SW_ACCESS  component=Tmeasy  system_inst=4  parameter=HCI
  SW_Vehicle_1_HCI : dyna_cpt_lib/CPT_MDL_HCI_SW_ACCESS  Tag=vedynaCPT_MDL_HCI_SW_ACCESS  component=Vehicle  system_inst=1  parameter=HCI
  SW_Wheel_1_HCI : dyna_cpt_lib/CPT_MDL_HCI_SW_ACCESS  Tag=vedynaCPT_MDL_HCI_SW_ACCESS  component=Wheel  system_inst=1  parameter=HCI
  SW_Wheel_2_HCI : dyna_cpt_lib/CPT_MDL_HCI_SW_ACCESS  Tag=vedynaCPT_MDL_HCI_SW_ACCESS  component=Wheel  system_inst=2  parameter=HCI
  SW_Wheel_3_HCI : dyna_cpt_lib/CPT_MDL_HCI_SW_ACCESS  Tag=vedynaCPT_MDL_HCI_SW_ACCESS  component=Wheel  system_inst=3  parameter=HCI
  SW_Wheel_4_HCI : dyna_cpt_lib/CPT_MDL_HCI_SW_ACCESS  Tag=vedynaCPT_MDL_HCI_SW_ACCESS  component=Wheel  system_inst=4  parameter=HCI
  Tmeasy_{5..6,9..14} (8 alike) : Ground
  Wheel_{5..6,9..14} (8 alike) : Ground
  HCI Switches : Outport
  wires:
  Tmeasy_14/1 -> Mux/27
  Tmeasy_13/1 -> Mux/25
  Wheel_14/1 -> Mux/28
  Wheel_13/1 -> Mux/26
  Wheel_12/1 -> Mux/24
  Tmeasy_12/1 -> Mux/23
  Wheel_11/1 -> Mux/22
  Tmeasy_11/1 -> Mux/21
  Wheel_10/1 -> Mux/20
  Tmeasy_10/1 -> Mux/19
  Wheel_9/1 -> Mux/18
  Tmeasy_9/1 -> Mux/17
  Wheel_6/1 -> Mux/16
  Tmeasy_6/1 -> Mux/15
  Wheel_5/1 -> Mux/14
  Tmeasy_5/1 -> Mux/13
  SW_Wheel_4_HCI/1 -> Mux/12
  SW_Tmeasy_4_HCI/1 -> Mux/11
  SW_Wheel_3_HCI/1 -> Mux/10
  SW_Tmeasy_3_HCI/1 -> Mux/9
  SW_Wheel_2_HCI/1 -> Mux/8
  SW_Tmeasy_2_HCI/1 -> Mux/7
  SW_Wheel_1_HCI/1 -> Mux/6
  SW_Tmeasy_1_HCI/1 -> Mux/5
  SW_Driveline_1_HCI/1 -> Mux/4
  SW_Engine_1_HCI/1 -> Mux/3
  SW_Chassis_1_HCI/1 -> Mux/2
  SW_Vehicle_1_HCI/1 -> Mux/1
  Mux/1 -> HCI Switches/1

== system Demo_veDYNA_cs/Vedyna_Vehicle/vdy_mdl/Vehicle System/veDYNA Vehicle Subsystem/Maneuver Commands Splitter ==
  note: veDYNA Maneuver Command Splitter
  note: COPYRIGHT 2002 by TESIS DYNAware GmbH
  SyncIn : Inport
  Maneuver Commands : Inport  Port=2
  Demux : Demux  Outputs=[1,8,9]
  SyncOut : Outport
  Maneuver Commands to External Inputs : Outport  Port=2
  Maneuver Commands to Brake System : Outport  Port=3
  Maneuver Commands to Vehicle : Outport  Port=4
  wires:
  SyncIn/1 -> SyncOut/1
  Maneuver Commands/1 -> Demux/1
  Demux/3 -> Maneuver Commands to External Inputs/1
  Demux/1 -> Maneuver Commands to Brake System/1
  Demux/2 -> Maneuver Commands to Vehicle/1

== system Demo_veDYNA_cs/Vedyna_Vehicle/vdy_mdl/Vehicle System/veDYNA Vehicle Subsystem/Vehicle Outputs to I/O ==
  note: COPYRIGHT 2002 by TESIS DYNAware GmbH
  note: veDYNA Vehicle Interface to I/O (optional)
  SyncIn : Inport
  Read From WorkSpace : dyna_lib/Read From WorkSpace  comp=Wheel|Wheel|Wheel|Wheel|Wheel|Wheel|Wheel|Wheel  inst=0|1|2|3|4|5|6|7  group=wheelstate_v|wheelstate_v|wheelstate_v|wheelstate_v|wheelstate_v|wheelstate_v|wheelstate_v|wheelstate_v  var=or|or|or|or|or|or|or|or
  Output to IO : Outport
  SyncOut : Outport  Port=2
  wires:
  SyncIn/1 -> SyncOut/1
  Read From WorkSpace/1 -> Output to IO/1

== system Demo_veDYNA_cs/BMW_X5_1/Trajectories/Traj2State1/Traj2State2/Traj2MuxState_Ext/demux ==
  traj : Inport
  Demux : Demux  Outputs=18
  x : Outport
  y : Outport  Port=2
  z : Outport  Port=3
  velx : Outport  Port=4
  vely : Outport  Port=5
  velz : Outport  Port=6
  R : Outport  Port=7
  P : Outport  Port=8
  Y : Outport  Port=9
  velR : Outport  Port=10
  velP : Outport  Port=11
  velY : Outport  Port=12
  accx : Outport  Port=13
  accy : Outport  Port=14
  accz : Outport  Port=15
  accR : Outport  Port=16
  accP : Outport  Port=17
  accY : Outport  Port=18
  wires:
  Demux/18 -> accY/1
  Demux/17 -> accP/1
  Demux/16 -> accR/1
  Demux/15 -> accz/1
  Demux/14 -> accy/1
  Demux/13 -> accx/1
  Demux/12 -> velY/1
  Demux/11 -> velP/1
  Demux/10 -> velR/1
  Demux/9 -> velz/1
  Demux/8 -> vely/1
  Demux/7 -> velx/1
  Demux/6 -> Y/1
  Demux/5 -> P/1
  traj/1 -> Demux/1
  Demux/4 -> R/1
  Demux/3 -> z/1
  Demux/2 -> y/1
  Demux/1 -> x/1

== system Demo_veDYNA_cs/Nissan_Cabstar_1/Trajectories/Traj2State1/Traj2State2/Traj2MuxState_Ext/demux ==
  traj : Inport
  Demux : Demux  Outputs=18
  x : Outport
  y : Outport  Port=2
  z : Outport  Port=3
  velx : Outport  Port=4
  vely : Outport  Port=5
  velz : Outport  Port=6
  R : Outport  Port=7
  P : Outport  Port=8
  Y : Outport  Port=9
  velR : Outport  Port=10
  velP : Outport  Port=11
  velY : Outport  Port=12
  accx : Outport  Port=13
  accy : Outport  Port=14
  accz : Outport  Port=15
  accR : Outport  Port=16
  accP : Outport  Port=17
  accY : Outport  Port=18
  wires:
  Demux/18 -> accY/1
  Demux/17 -> accP/1
  Demux/16 -> accR/1
  Demux/15 -> accz/1
  Demux/14 -> accy/1
  Demux/13 -> accx/1
  Demux/12 -> velY/1
  Demux/11 -> velP/1
  Demux/10 -> velR/1
  Demux/9 -> velz/1
  Demux/8 -> vely/1
  Demux/7 -> velx/1
  Demux/6 -> Y/1
  Demux/5 -> P/1
  traj/1 -> Demux/1
  Demux/4 -> R/1
  Demux/3 -> z/1
  Demux/2 -> y/1
  Demux/1 -> x/1

== system Demo_veDYNA_cs/Vedyna_Vehicle/CPT_MDL/MDL_PAR/BrkHyd/System Instance 1/pbrmaster [N/m**2] ==
  Table : Lookup  InputValues=CPT.MDL_PAR.BrkHyd{1}.pbrmaster.Table.x  Table=CPT.MDL_PAR.BrkHyd{1}.pbrmaster.Table.v  SaturateOnIntegerOverflow=on
  Terminator : Terminator
  Terminator1 : Terminator
  Value : Constant  Value=CPT.MDL_PAR.BrkHyd{1}.pbrmaster.Value.v
  tag scope: BrkHyd_1_pbrmaster_TBL=global, BrkHyd_1_pbrmaster_VAL=global
  wires:
  [vdy_Simctrl_tsim] -> Table/1
  Value/1 -> [BrkHyd_1_pbrmaster_VAL]
  [BrkHyd_1_pbrmaster_VAL] -> Terminator/1
  [BrkHyd_1_pbrmaster_TBL] -> Terminator1/1
  Table/1 -> [BrkHyd_1_pbrmaster_TBL]

== system Demo_veDYNA_cs/Vedyna_Vehicle/CPT_MDL/MDL_PAR/ClutchCtrl/System Instance 1/Clutch [%] ==
  Table : Lookup  InputValues=CPT.MDL_PAR.ClutchCtrl{1}.Clutch.Table.x  Table=CPT.MDL_PAR.ClutchCtrl{1}.Clutch.Table.v  SaturateOnIntegerOverflow=on
  Terminator : Terminator
  Terminator1 : Terminator
  Value : Constant  Value=CPT.MDL_PAR.ClutchCtrl{1}.Clutch.Value.v
  tag scope: ClutchCtrl_1_Clutch_TBL=global, ClutchCtrl_1_Clutch_VAL=global
  wires:
  [vdy_Simctrl_tsim] -> Table/1
  Value/1 -> [ClutchCtrl_1_Clutch_VAL]
  [ClutchCtrl_1_Clutch_VAL] -> Terminator/1
  [ClutchCtrl_1_Clutch_TBL] -> Terminator1/1
  Table/1 -> [ClutchCtrl_1_Clutch_TBL]

== system Demo_veDYNA_cs/Vedyna_Vehicle/CPT_MDL/MDL_PAR/Contact/System Instance 1/RoadZ [m] ==
  Table : Lookup  InputValues=CPT.MDL_PAR.Contact{1}.RoadZ.Table.x  Table=CPT.MDL_PAR.Contact{1}.RoadZ.Table.v  SaturateOnIntegerOverflow=on
  Terminator : Terminator
  Terminator1 : Terminator
  Value : Constant  Value=CPT.MDL_PAR.Contact{1}.RoadZ.Value.v
  tag scope: Contact_1_RoadZ_TBL=global, Contact_1_RoadZ_VAL=global
  wires:
  [vdy_Simctrl_tsim] -> Table/1
  Value/1 -> [Contact_1_RoadZ_VAL]
  [Contact_1_RoadZ_VAL] -> Terminator/1
  [Contact_1_RoadZ_TBL] -> Terminator1/1
  Table/1 -> [Contact_1_RoadZ_TBL]

== system Demo_veDYNA_cs/Vedyna_Vehicle/CPT_MDL/MDL_PAR/Contact/System Instance 2/RoadZ [m] ==
  Table : Lookup  InputValues=CPT.MDL_PAR.Contact{2}.RoadZ.Table.x  Table=CPT.MDL_PAR.Contact{2}.RoadZ.Table.v  SaturateOnIntegerOverflow=on
  Terminator : Terminator
  Terminator1 : Terminator
  Value : Constant  Value=CPT.MDL_PAR.Contact{2}.RoadZ.Value.v
  tag scope: Contact_2_RoadZ_TBL=global, Contact_2_RoadZ_VAL=global
  wires:
  [vdy_Simctrl_tsim] -> Table/1
  Value/1 -> [Contact_2_RoadZ_VAL]
  [Contact_2_RoadZ_VAL] -> Terminator/1
  [Contact_2_RoadZ_TBL] -> Terminator1/1
  Table/1 -> [Contact_2_RoadZ_TBL]

== system Demo_veDYNA_cs/Vedyna_Vehicle/CPT_MDL/MDL_PAR/Contact/System Instance 3/RoadZ [m] ==
  Table : Lookup  InputValues=CPT.MDL_PAR.Contact{3}.RoadZ.Table.x  Table=CPT.MDL_PAR.Contact{3}.RoadZ.Table.v  SaturateOnIntegerOverflow=on
  Terminator : Terminator
  Terminator1 : Terminator
  Value : Constant  Value=CPT.MDL_PAR.Contact{3}.RoadZ.Value.v
  tag scope: Contact_3_RoadZ_TBL=global, Contact_3_RoadZ_VAL=global
  wires:
  [vdy_Simctrl_tsim] -> Table/1
  Value/1 -> [Contact_3_RoadZ_VAL]
  [Contact_3_RoadZ_VAL] -> Terminator/1
  [Contact_3_RoadZ_TBL] -> Terminator1/1
  Table/1 -> [Contact_3_RoadZ_TBL]

== system Demo_veDYNA_cs/Vedyna_Vehicle/CPT_MDL/MDL_PAR/Contact/System Instance 4/RoadZ [m] ==
  Table : Lookup  InputValues=CPT.MDL_PAR.Contact{4}.RoadZ.Table.x  Table=CPT.MDL_PAR.Contact{4}.RoadZ.Table.v  SaturateOnIntegerOverflow=on
  Terminator : Terminator
  Terminator1 : Terminator
  Value : Constant  Value=CPT.MDL_PAR.Contact{4}.RoadZ.Value.v
  tag scope: Contact_4_RoadZ_TBL=global, Contact_4_RoadZ_VAL=global
  wires:
  [vdy_Simctrl_tsim] -> Table/1
  Value/1 -> [Contact_4_RoadZ_VAL]
  [Contact_4_RoadZ_VAL] -> Terminator/1
  [Contact_4_RoadZ_TBL] -> Terminator1/1
  Table/1 -> [Contact_4_RoadZ_TBL]

== system Demo_veDYNA_cs/Vedyna_Vehicle/CPT_MDL/MDL_PAR/Contact/System Instance 5/RoadZ [m] ==
  Table : Lookup  InputValues=CPT.MDL_PAR.Contact{5}.RoadZ.Table.x  Table=CPT.MDL_PAR.Contact{5}.RoadZ.Table.v  SaturateOnIntegerOverflow=on
  Terminator : Terminator
  Terminator1 : Terminator
  Value : Constant  Value=CPT.MDL_PAR.Contact{5}.RoadZ.Value.v
  tag scope: Contact_5_RoadZ_TBL=global, Contact_5_RoadZ_VAL=global
  wires:
  [vdy_Simctrl_tsim] -> Table/1
  Value/1 -> [Contact_5_RoadZ_VAL]
  [Contact_5_RoadZ_VAL] -> Terminator/1
  [Contact_5_RoadZ_TBL] -> Terminator1/1
  Table/1 -> [Contact_5_RoadZ_TBL]

== system Demo_veDYNA_cs/Vedyna_Vehicle/CPT_MDL/MDL_PAR/Contact/System Instance 6/RoadZ [m] ==
  Table : Lookup  InputValues=CPT.MDL_PAR.Contact{6}.RoadZ.Table.x  Table=CPT.MDL_PAR.Contact{6}.RoadZ.Table.v  SaturateOnIntegerOverflow=on
  Terminator : Terminator
  Terminator1 : Terminator
  Value : Constant  Value=CPT.MDL_PAR.Contact{6}.RoadZ.Value.v
  tag scope: Contact_6_RoadZ_TBL=global, Contact_6_RoadZ_VAL=global
  wires:
  [vdy_Simctrl_tsim] -> Table/1
  Value/1 -> [Contact_6_RoadZ_VAL]
  [Contact_6_RoadZ_VAL] -> Terminator/1
  [Contact_6_RoadZ_TBL] -> Terminator1/1
  Table/1 -> [Contact_6_RoadZ_TBL]

== system Demo_veDYNA_cs/Vedyna_Vehicle/CPT_MDL/MDL_PAR/Contact/System Instance 7/RoadZ [m] ==
  Table : Lookup  InputValues=CPT.MDL_PAR.Contact{7}.RoadZ.Table.x  Table=CPT.MDL_PAR.Contact{7}.RoadZ.Table.v  SaturateOnIntegerOverflow=on
  Terminator : Terminator
  Terminator1 : Terminator
  Value : Constant  Value=CPT.MDL_PAR.Contact{7}.RoadZ.Value.v
  tag scope: Contact_7_RoadZ_TBL=global, Contact_7_RoadZ_VAL=global
  wires:
  [vdy_Simctrl_tsim] -> Table/1
  Value/1 -> [Contact_7_RoadZ_VAL]
  [Contact_7_RoadZ_VAL] -> Terminator/1
  [Contact_7_RoadZ_TBL] -> Terminator1/1
  Table/1 -> [Contact_7_RoadZ_TBL]

== system Demo_veDYNA_cs/Vedyna_Vehicle/CPT_MDL/MDL_PAR/Contact/System Instance 8/RoadZ [m] ==
  Table : Lookup  InputValues=CPT.MDL_PAR.Contact{8}.RoadZ.Table.x  Table=CPT.MDL_PAR.Contact{8}.RoadZ.Table.v  SaturateOnIntegerOverflow=on
  Terminator : Terminator
  Terminator1 : Terminator
  Value : Constant  Value=CPT.MDL_PAR.Contact{8}.RoadZ.Value.v
  tag scope: Contact_8_RoadZ_TBL=global, Contact_8_RoadZ_VAL=global
  wires:
  [vdy_Simctrl_tsim] -> Table/1
  Value/1 -> [Contact_8_RoadZ_VAL]
  [Contact_8_RoadZ_VAL] -> Terminator/1
  [Contact_8_RoadZ_TBL] -> Terminator1/1
  Table/1 -> [Contact_8_RoadZ_TBL]

== system Demo_veDYNA_cs/Vedyna_Vehicle/CPT_MDL/MDL_PAR/Driver/System Instance 1/acc_comp_scale [-] ==
  Table : Lookup  InputValues=CPT.MDL_PAR.Driver{1}.acc_comp_scale.Table.x  Table=CPT.MDL_PAR.Driver{1}.acc_comp_scale.Table.v  SaturateOnIntegerOverflow=on
  Terminator : Terminator
  Terminator1 : Terminator
  Value : Constant  Value=CPT.MDL_PAR.Driver{1}.acc_comp_scale.Value.v
  tag scope: Driver_1_acc_comp_scale_TBL=global, Driver_1_acc_comp_scale_VAL=global
  wires:
  [vdy_Simctrl_tsim] -> Table/1
  Value/1 -> [Driver_1_acc_comp_scale_VAL]
  [Driver_1_acc_comp_scale_VAL] -> Terminator/1
  [Driver_1_acc_comp_scale_TBL] -> Terminator1/1
  Table/1 -> [Driver_1_acc_comp_scale_TBL]

== system Demo_veDYNA_cs/Vedyna_Vehicle/CPT_MDL/MDL_PAR/Driver/System Instance 1/adj_acc_gain [-] ==
  Table : Lookup  InputValues=CPT.MDL_PAR.Driver{1}.adj_acc_gain.Table.x  Table=CPT.MDL_PAR.Driver{1}.adj_acc_gain.Table.v  SaturateOnIntegerOverflow=on
  Terminator : Terminator
  Terminator1 : Terminator
  Value : Constant  Value=CPT.MDL_PAR.Driver{1}.adj_acc_gain.Value.v
  tag scope: Driver_1_adj_acc_gain_TBL=global, Driver_1_adj_acc_gain_VAL=global
  wires:
  [vdy_Simctrl_tsim] -> Table/1
  Value/1 -> [Driver_1_adj_acc_gain_VAL]
  [Driver_1_adj_acc_gain_VAL] -> Terminator/1
  [Driver_1_adj_acc_gain_TBL] -> Terminator1/1
  Table/1 -> [Driver_1_adj_acc_gain_TBL]

== system Demo_veDYNA_cs/Vedyna_Vehicle/CPT_MDL/MDL_PAR/Driver/System Instance 1/adj_brake_gain [-] ==
  Table : Lookup  InputValues=CPT.MDL_PAR.Driver{1}.adj_brake_gain.Table.x  Table=CPT.MDL_PAR.Driver{1}.adj_brake_gain.Table.v  SaturateOnIntegerOverflow=on
  Terminator : Terminator
  Terminator1 : Terminator
  Value : Constant  Value=CPT.MDL_PAR.Driver{1}.adj_brake_gain.Value.v
  tag scope: Driver_1_adj_brake_gain_TBL=global, Driver_1_adj_brake_gain_VAL=global
  wires:
  [vdy_Simctrl_tsim] -> Table/1
  Value/1 -> [Driver_1_adj_brake_gain_VAL]
  [Driver_1_adj_brake_gain_VAL] -> Terminator/1
  [Driver_1_adj_brake_gain_TBL] -> Terminator1/1
  Table/1 -> [Driver_1_adj_brake_gain_TBL]

== system Demo_veDYNA_cs/Vedyna_Vehicle/CPT_MDL/MDL_PAR/Driver/System Instance 1/ax_min [m/s^2] ==
  Table : Lookup  InputValues=CPT.MDL_PAR.Driver{1}.ax_min.Table.x  Table=CPT.MDL_PAR.Driver{1}.ax_min.Table.v  SaturateOnIntegerOverflow=on
  Terminator : Terminator
  Terminator1 : Terminator
  Value : Constant  Value=CPT.MDL_PAR.Driver{1}.ax_min.Value.v
  tag scope: Driver_1_ax_min_TBL=global, Driver_1_ax_min_VAL=global
  wires:
  [vdy_Simctrl_tsim] -> Table/1
  Value/1 -> [Driver_1_ax_min_VAL]
  [Driver_1_ax_min_VAL] -> Terminator/1
  [Driver_1_ax_min_TBL] -> Terminator1/1
  Table/1 -> [Driver_1_ax_min_TBL]

== system Demo_veDYNA_cs/Vedyna_Vehicle/CPT_MDL/MDL_PAR/Driver/System Instance 1/ctrl_acc_smooth_t [s] ==
  Table : Lookup  InputValues=CPT.MDL_PAR.Driver{1}.ctrl_acc_smooth_t.Table.x  Table=CPT.MDL_PAR.Driver{1}.ctrl_acc_smooth_t.Table.v  SaturateOnIntegerOverflow=on
  Terminator : Terminator
  Terminator1 : Terminator
  Value : Constant  Value=CPT.MDL_PAR.Driver{1}.ctrl_acc_smooth_t.Value.v
  tag scope: Driver_1_ctrl_acc_smooth_t_TBL=global, Driver_1_ctrl_acc_smooth_t_VAL=global
  wires:
  [vdy_Simctrl_tsim] -> Table/1
  Value/1 -> [Driver_1_ctrl_acc_smooth_t_VAL]
  [Driver_1_ctrl_acc_smooth_t_VAL] -> Terminator/1
  [Driver_1_ctrl_acc_smooth_t_TBL] -> Terminator1/1
  Table/1 -> [Driver_1_ctrl_acc_smooth_t_TBL]

== system Demo_veDYNA_cs/Vedyna_Vehicle/CPT_MDL/MDL_PAR/Driver/System Instance 1/cu_comp_scale [-] ==
  Table : Lookup  InputValues=CPT.MDL_PAR.Driver{1}.cu_comp_scale.Table.x  Table=CPT.MDL_PAR.Driver{1}.cu_comp_scale.Table.v  SaturateOnIntegerOverflow=on
  Terminator : Terminator
  Terminator1 : Terminator
  Value : Constant  Value=CPT.MDL_PAR.Driver{1}.cu_comp_scale.Value.v
  tag scope: Driver_1_cu_comp_scale_TBL=global, Driver_1_cu_comp_scale_VAL=global
  wires:
  [vdy_Simctrl_tsim] -> Table/1
  Value/1 -> [Driver_1_cu_comp_scale_VAL]
  [Driver_1_cu_comp_scale_VAL] -> Terminator/1
  [Driver_1_cu_comp_scale_TBL] -> Terminator1/1
  Table/1 -> [Driver_1_cu_comp_scale_TBL]

== system Demo_veDYNA_cs/Vedyna_Vehicle/CPT_MDL/MDL_PAR/Driver/System Instance 1/cu_path [1/m] ==
  Table : Lookup  InputValues=CPT.MDL_PAR.Driver{1}.cu_path.Table.x  Table=CPT.MDL_PAR.Driver{1}.cu_path.Table.v  SaturateOnIntegerOverflow=on
  Terminator : Terminator
  Terminator1 : Terminator
  Value : Constant  Value=CPT.MDL_PAR.Driver{1}.cu_path.Value.v
  tag scope: Driver_1_cu_path_TBL=global, Driver_1_cu_path_VAL=global
  wires:
  [vdy_Driver_s] -> Table/1
  Value/1 -> [Driver_1_cu_path_VAL]
  [Driver_1_cu_path_VAL] -> Terminator/1
  [Driver_1_cu_path_TBL] -> Terminator1/1
  Table/1 -> [Driver_1_cu_path_TBL]
